simulink model "KoopmanMPC"  (R2023b)
settings: Solver=FixedStepAuto  StartTime=0.0  StopTime=inf  FixedStep=0.01  RelTol=1e-3
values from neighbouring files (symbols this model uses):
  ref_resampled_4 = [-0.0434326850921 1.00739834805 -5.2965480502 -0.0275886266971 -0.00523965410955 0.0242941259565 0.000763390489614 -0.0605545134458 1.09554308151 -5.3213592223 -0.0277571536527 -0.0053597164637 ... (2807 elements, 7x401)]    [circle_resampled_trajectory_4.mat]
undefined symbols (not defined in the file or in its folder): canChannel
libraries: canmsglib x15, canlib x11, simulink x11, dspfdesign x7, auroraNDILibrary x1
(part 2 of 2)

== matlab function KoopmanMPC/Initial_flag=1/RandomControlSequence3 ==
  settings: updateMethod=DISCRETE
  data: u output; force_meas input; F_min input; F_max input; step input
function u = tension_control(force_meas,F_min,F_max,step)
    u_pull = step; % small constant torque or velocity
    u_relax = -step;
    
    if force_meas < F_min
        u = u_pull;
    elseif force_meas > F_max
        u = u_relax;
    else
        u = 0; % hold
    end
end

== matlab function KoopmanMPC/Displacement_mode_flag=2/Subsystem/MPC ==
  settings: updateMethod=DISCRETE  sampleTime=0.01
  data: pos input; predStep input; itLast input; u0_sc input; yMotor output; zMotor output; debug output; realState output; yHorRec output; zHorRec output; uHor output size=[10 2]; it output; ref data_store_memory; c data_store_memory; D data_store_memory; G data_store_memory; H data_store_memory; L data_store_memory; M data_store_memory; uWarm_sc output; DelayEmbedState data_store_memory; DelayEmbedU data_store_memory
function [yMotor,zMotor,debug,realState,yHorRec,zHorRec,uHor,it,uWarm_sc]  = fcn(pos,predStep,itLast,u0_sc)
% Returns the calculated control action (required cable tension). They are
% the first control action from the calculated control sequence with MPC
% scheme.
%
% INPUT
% tip_pos_orie - vector of dimension (6,1) where the first element
%                represents the bending angle and the next two elements
%                represent the normolized bending direction projected to
%                the x-axis nd z-axis
% time - simulation time signal
% z_warm - initial guess of the decision variables which are stacked vertically as
%          a collected variables vector, consist of the state and control
%          variables and the slack variables z_warm = [u_warm^T, x_warm^T,
%          s_warm^T]^T
% u0_sc - initial gueess for the Quadprog solver, after normalization
%
% OUTPUT
% force_top  - required cable tension of the top cable, along with the
%              negative x-axis direction
% force_btm  - required cable tension of the bottom cable, along with the
%              positive x-axis direction
% force_right - required cable tension of the riht cable, along with the
%              positive z-axis direction
% force_left - required cable tension of the left cable, along with the
%              negative z-axis direction
% z_last   - the decision variables at last instance, used for warmstarting
%            the SQP.
% flag   - an integer that describes the exit condition of SQP. 1
%          represents function converged to the solution x within maximum iteration,
%          and 0 represents the SQP algorithm can not find a solution within maximum
%          iteration.
%
%
% Developed by Yongjun Yan. Updated July 21 2025.
global ref c D G H L M DelayEmbedU DelayEmbedState
%% Initialization
% Horizon = 0.2;
% Samp_time = 0.01; 
Num = predStep;
%% Read Sensor and Update the Global Variables
% pos = [x,y,z,q0,q1,q2,q3];
% DelayEmbedObs = [DelayEmbedObs(8:end);pos']; % DelayEmbedObs is 1*245

%% Solve the optimal control problem
preMtx.c = c;
preMtx.D = D;
preMtx.G = G;
preMtx.H = H;
preMtx.L = L;
preMtx.M = M;
params.horizon = Num;
params.nd = 1;
params.m = 2; % number of control variables
params.n = 7; % number of states
%% Get the position and velocity information (sequence) over the horizon
% get current state and input with delays
if itLast == 1
    y0 =  [ref(:,1),ref(:,1)] ;
    u0 = DelayEmbedU ;
    % initialize results struct
    % set initial condition
    initial.y = scaledown_y(y0'); initial.u = scaledown_u(u0');
    % zeta0 = get_zeta(params, initial );    % LINE NOT NEEDED
    % initialize results struct
    DelayEmbedState = y0;

    current.y = scaledown_y( y0' );   
    current.u = scaledown_u( u0' ); 
else
    y = DelayEmbedState;
    u = DelayEmbedU;
    current.y = scaledown_y( y' ); 
    current.u = scaledown_u( u' ); 
end
itLastRef = mod(itLast,400);
% isolate the reference trajectory over the horizon
% if itLast + Num <= 401
    refHor = ref(:, itLastRef+1:itLastRef + Num + 1);
% else
%     refHor = ref(:, itLast : end );     % repeat last entry
% end 

refHorLow = scaledown_y(refHor');
debug = size(refHorLow);
% construct the current value of zeta
zeta_temp = get_zeta(params, current );
zeta = zeta_temp( end , : )';   % want most recent points

% lift zeta
z = lift_full( zeta' );

%%
% vectorize the reference trajectory
Yr = reshape( refHorLow' , [ size(refHorLow,1)* size(refHorLow,2) , 1 ] );

% setup matrices for gurobi solverfile
H_qp = preMtx.H;     
f = ( z' * preMtx.G + Yr' * preMtx.D )';
A = preMtx.L;
b = - preMtx.M * z + preMtx.c;

% tack on "memory" constraint to fix initial input u_0
Atack = [ [ speye( params.m ) ; -speye( params.m ) ] , sparse( 2*params.m , size(A,2) - params.m ) ];
%             Atack_bot = [ sparse( 2*obj.params.m , obj.params.m) , [ speye( obj.params.m ) ; -speye( obj.params.m ) ] , sparse( 2*obj.params.m , size(A,2) - 2*obj.params.m ) ];
%             Atack = [ Atack_top ; Atack_bot ];
btack = [ current.u(end,:)' ; -current.u(end,:)' ];
A = full([A ; Atack]);    % tack on memory constraint
b = full([b ; btack]);

% solve the MPC problem
%             Uvec = quadprog_gurobi( H , f , A , b );   % solve using gurobi (returns NaNs of cannot be solved)

% % Define constants
% coder.cinclude("xpcimports.h");
% 
% % Declare and assign using opaque
% t_start = coder.ceval('xpcTargetTimerTickCount');

options = optimoptions('quadprog','Algorithm','active-set','MaxIterations',3000);
% % options = optimoptions(options,'MaxIterations',30);
% 
x0 = u0_sc;
Uvec = quadprog(2*H_qp,f,A,b,[],[],[],[],x0,options);
% Uvec = zeros(20,1);

% Uvec = quadprog( 2*H , f , A , b );     % solve using matlab

% t_end = coder.ceval('xpcTargetTimerTickCount');
% tick_period = coder.ceval('xpcTargetTimerPeriod');
% 
% % Compute time in seconds
% solve_time = double(t_end - t_start) * double(tick_period);

% reshape the output so each input will have one row (first row equals current input)

U = reshape( Uvec ,  params.m , Num  );
uHor = zeros(10, 2);
uHor(1:10, :) = scaleup_u( U');

% isolate input for this step (may need to make it U(1,:)
u_kp1_sc = U( : , 2 );

% scaleup the input for the results
u_kp1 = scaleup_u( u_kp1_sc' );

% simulate the system over one time-step
z_k = z;
u_k_sc = scaledown_u( DelayEmbedU(:,2)' );  % need to use previously calculated input NEED TO MAKE THIS CLEANER!!!

y_kp1 = ref(:,1);  % Initialize with reference point
yHorRec = zeros(7,11);
zHorRec = zeros(19,11);
yHorRec(:,1) = scaledown_y(DelayEmbedState(:,2)');
zHorRec(:,1) = z_k;
for i = 1:Num
    if i == 1
        zHorRec(:,2) = valf( zHorRec(:,1)' , u_k_sc);
        yHorRec(:,2) = D_lowDim(zHorRec(:,2)');
        y_kp1 = scaleup_y( yHorRec(:,2)' )';  % scale output back up 
    else
        zHorRec(:,i+1) = valf( zHorRec(:,i)' , U( : , i )');
        yHorRec(:,i+1) = D_lowDim(zHorRec(:,i+1)');
        % y_kp1 = scaleup_y( yHorRec(:,i+1)' )';  % scale output back up 
    end
end
% record updated results
DelayEmbedU = [DelayEmbedU(:,2), u_kp1'];
DelayEmbedState = [DelayEmbedState(:,2),pos'];
realState = y_kp1;
yMotor = u_k_sc(1);
zMotor = u_k_sc(2);
uWarm_sc = Uvec;
               
it = itLast + 1;
%% for debug
% yMotor = 1;
% zMotor = 1;
% uWarm_sc = zeros(40,1);
% debug = size(z);
end

== matlab function KoopmanMPC/Displacement_mode_flag=2/MATLAB Function ==
  data: yMotorNorm input; Motor1 output; zMotorNorm input; Motor2 output; Motor3 output; Motor4 output
function [Motor1,Motor2,Motor3,Motor4] = allocation(yMotorNorm,zMotorNorm)

uScaledUp = scaleup_u([yMotorNorm,zMotorNorm]);
yMotor = uScaledUp(1);
zMotor = uScaledUp(2);

retractionrFactor = 2;
if yMotor > 0
    Motor2 = yMotor;
    Motor3 = -retractionrFactor*yMotor;
else
    Motor2 = retractionrFactor*yMotor;
    Motor3 = -yMotor;
end

if zMotor > 0
    Motor4 = zMotor;
    Motor1 = -retractionrFactor*zMotor;
else
    Motor4 = retractionrFactor*zMotor;
    Motor1 = -zMotor;
end

end

== matlab function KoopmanMPC/MATLAB Function11 ==
  data: y output; u input; u_last input
function y = fcn(u,u_last)
if abs(u-u_last)>200
    y = u_last;
else
    y = u;
end

== matlab function KoopmanMPC/Displacement_mode_flag=2/MATLAB Function1 ==
  data: pos_x input; Pos_rel output; pos_y input; Pos0 output size=[1,7]; it output; pos_z input; q0 input; q1 input; q2 input; q3 input; Pos0Last input; itLast input
function [Pos_rel,Pos0,it] = allocation(pos_x,pos_y,pos_z,q0,q1,q2,q3,Pos0Last,itLast)
Pos_now = [pos_x,pos_y,pos_z,q0,q1,q2,q3];
if itLast == 1
    Pos0 = Pos_now;
else
    Pos0 = Pos0Last';
end

Pos_rel = Pos_now - Pos0;
it = itLast + 1;
end
